simulink model "impulse_ex_3_b"  (R2024a)
settings: Solver=VariableStepAuto  StartTime=0.0  StopTime=6.23456  RelTol=1e-6  AbsTol=1e-6
values from neighbouring files (symbols this model uses):
  a = 0.001    [impulseDD.sldd]
undefined symbols (not defined in the file or in its folder): Call, Function, sys
libraries: simulink x1
settings Model: DataDictionary=impulseDD.sldd  Creator=grouleau  LastModifiedBy=grouleau

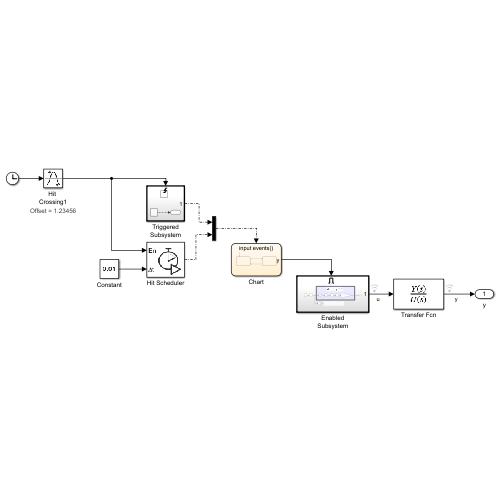
[thumbnail: Simulink's stored preview of the top-level diagram]
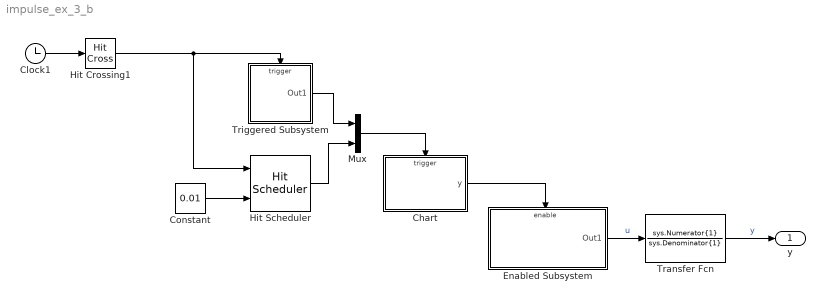
== system impulse_ex_3_b ==
  Chart : Stateflow chart  TreatAsAtomicUnit=on
  Clock1 : Clock
  Constant : Constant  Value=0.01
  Enabled Subsystem : Subsystem  TreatAsAtomicUnit=on
  Hit Crossing1 : HitCross  HitCrossingOffset=1.23456
      settings: AttributesFormatString=Offset = %<HitCrossingOffset>
  Hit Scheduler : HitScheduler  HitSchedulerOutputType=Function-Call
  Mux : Mux  Inputs=2
  Transfer Fcn : TransferFcn  Numerator=sys.Numerator{1}  Denominator=sys.Denominator{1}
  Triggered Subsystem : Subsystem  TreatAsAtomicUnit=on
  y : Outport
  wires:
  Transfer Fcn/1 -> y/1  "y"
  Enabled Subsystem/1(Out1) -> Transfer Fcn/1  "u"
  Mux/1 -> Chart/Trigger
  Constant/1 -> Hit Scheduler/2
  Triggered Subsystem/1(Out1) -> Mux/1
  Hit Scheduler/1 -> Mux/2
  Clock1/1 -> Hit Crossing1/1
  Chart/1(y) -> Enabled Subsystem/Enable
  Hit Crossing1/1 -> Hit Scheduler/1, Triggered Subsystem/Trigger

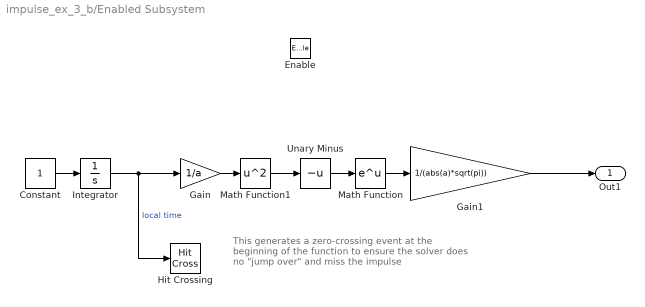
== system impulse_ex_3_b/Enabled Subsystem ==
  note: This generates a zero-crossing event at the beginning of the function to ensure the solver does no "jump over" and miss the impulse
  Enable : EnablePort  StatesWhenEnabling=reset
  Constant : Constant
  Gain : Gain  Gain=1/a
  Gain1 : Gain  Gain=1/(abs(a)*sqrt(pi))
  Hit Crossing : HitCross  HitCrossingOffset=-0.004  ShowOutputPort=off
  Integrator : Integrator  InitialCondition=-0.005
  Math Function : Math
  Math Function1 : Math  Operator=square
  Unary Minus : UnaryMinus
  Out1 : Outport  OutputWhenDisabled=reset  InitialOutput=0
  wires:
  Integrator/1 -> Hit Crossing/1, Gain/1  "local time"
  Math Function1/1 -> Unary Minus/1
  Math Function/1 -> Gain1/1
  Gain1/1 -> Out1/1
  Gain/1 -> Math Function1/1
  Unary Minus/1 -> Math Function/1
  Constant/1 -> Integrator/1

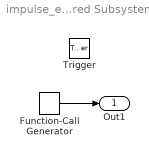
== system impulse_ex_3_b/Triggered Subsystem ==
  Trigger : TriggerPort  VariantControl=(inherit)
  Function-Call Generator : simulink/Ports & Subsystems/Function-Call Generator  sample_time=-1  numberOfIterations=1  DisallowWideOutput=off
  Out1 : Outport
  wires:
  Function-Call Generator/1 -> Out1/1

== stateflow chart impulse_ex_3_b/Chart ==
  settings: executeAtInitialization=1
  state off
    en:y=0;
  state on
    en: y=1/dt;
  (default) -> off
  off -> on : TrigOn
  on -> off : TrigOff
  data: y output; dt parameter
  events: TrigOn input FUNCTION_CALL_EVENT; TrigOff input FUNCTION_CALL_EVENT
